simulink model "l5"  (R2024a)
settings: Solver=FixedStepAuto  StartTime=0.0  StopTime=inf  RelTol=1e-3
libraries: robotlib x4
settings Model: Creator=ZY395  LastModifiedBy=ZY395
settings OptimizationCC: EnhancedBackFolding=on  PassReuseOutputArgsAs=Individual arguments  ZeroExternalMemoryAtStartup=off  ZeroInternalMemoryAtStartup=off  MaxStackSize=64  OptimizeBlockOrder=speed  DifferentSizesBufferReuse=on  OptimizationCustomize=off  EfficientTunableParamExpr=on
settings DebuggingCC: ParameterTunabilityLossMsg=error
settings HardwareCC: ProdBitPerPointer=32  ProdBitPerSizeT=32  ProdBitPerPtrDiffT=32  ProdLargestAtomicFloat=None  ProdIntDivRoundTo=Undefined  ProdEndianess=Unspecified  ProdWordSize=32  ProdHWDeviceType=Generic->Unspecified (assume 32-bit Generic)
settings SFSimCC: MATLABDynamicMemAlloc=off
settings RTWCC: Description=Embedded Coder  SystemTargetFile=ert.tlc  HardwareBoard=Robot Operating System (ROS)  TLCOptions="-aInlineSetEventsForThisBaseRateFcn=TLC_FALSE -aSuppressMultiTaskScheduler=TLC_FALSE  -aRateBasedStepFcn=0"  TemplateMakefile=ert_default_tmf  Toolchain=Catkin  TargetLang=C++
settings CodeAppCC: ForceParamTrailComments=on  IgnoreCustomStorageClasses=off  OperatorAnnotations=on  SimulinkDataObjDesc=on  SFDataObjDesc=on  InsertBlockDesc=on
settings ERTTargetCC: SupportContinuousTime=on  SupportNonInlinedSFcns=on

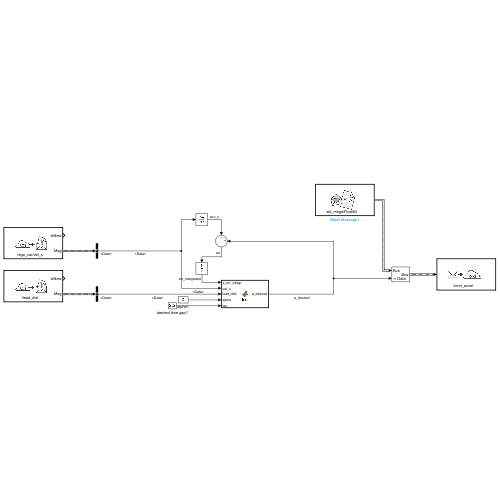
[thumbnail: Simulink's stored preview of the top-level diagram]
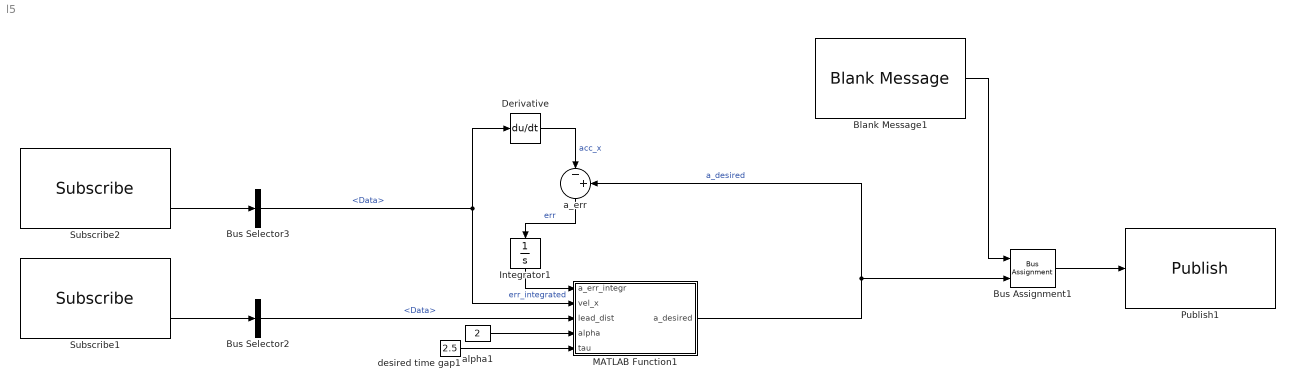
== system l5 ==
  Blank Message1 : robotlib/Blank Message  messageClass=Message  entityType=std_msgs/Float64  messageType=std_msgs/Float64  SampleTime=inf  legacyBusStruct=off
  Bus Assignment1 : BusAssignment  AssignedSignals=Data
  Bus Selector2 : BusSelector  OutputSignals=Data
  Bus Selector3 : BusSelector  OutputSignals=Data
  Derivative : Derivative
  Integrator1 : Integrator
  MATLAB Function1 : MATLAB Function  TreatAsAtomicUnit=on
  Publish1 : robotlib/Publish  topicSource=Specify your own  topic=/cmd_accel  messageType=std_msgs/Float64  legacyBusStruct=off  messageQueueLength=1
  Subscribe1 : robotlib/Subscribe  topicSource=Specify your own  topic=/lead_dist  messageType=std_msgs/Float64  SampleTime=-1  legacyBusStruct=off  messageQueueLength=1
  Subscribe2 : robotlib/Subscribe  topicSource=Specify your own  topic=/ego_car/vel_x  messageType=std_msgs/Float64  SampleTime=-1  legacyBusStruct=off  messageQueueLength=1
  a_err : Sum  Inputs=|-+
  alpha1 : Constant  Value=2
  desired time gap1 : Constant  Value=2.5
  wires:
  Blank Message1/1 -> Bus Assignment1/1
  Bus Assignment1/1 -> Publish1/1
  Bus Selector2/1 -> MATLAB Function1/3(lead_dist)  "<Data>"
  Subscribe1/2 -> Bus Selector2/1
  Subscribe2/2 -> Bus Selector3/1
  Derivative/1 -> a_err/1  "acc_x"
  Integrator1/1 -> MATLAB Function1/1(a_err_integr)  "err_integrated"
  a_err/1 -> Integrator1/1  "err"
  MATLAB Function1/1(a_desired) -> a_err/2, Bus Assignment1/2  "a_desired"
  alpha1/1 -> MATLAB Function1/4(alpha)
  Bus Selector3/1 -> Derivative/1, MATLAB Function1/2(vel_x)  "<Data>"
  desired time gap1/1 -> MATLAB Function1/5(tau)

== matlab function l5/MATLAB Function1 ==
  data: a_err_integr input; vel_x input; lead_dist input; a_desired output; alpha input; tau input
function a_desired = fcn(a_err_integr, vel_x, lead_dist, alpha, tau)
delt_tau = 0.5
tau_max = tau+delt_tau
tau_min = tau-delt_tau

time_gap = lead_dist/vel_x
a = alpha*(lead_dist - tau*vel_x)-1.5*a_err_integr;
if time_gap<tau_max && time_gap>tau_min
    ratio = abs(time_gap-tau)/delt_tau
    %a=a*(exp(ratio)-1)/(exp(1)-1)
    a=0.1*a
end

maxa=1.5;
mina=-3;
a_desired = min(max(mina,a), maxa);
